simulink model "WindTurbine_FireProtection_System"  (R2024b)
settings: Solver=ode4  StartTime=0.0  StopTime=60  FixedStep=0.1  RelTol=1e-3
libraries: simulink x3
settings Model: Creator=LENOVO  LastModifiedBy=LENOVO

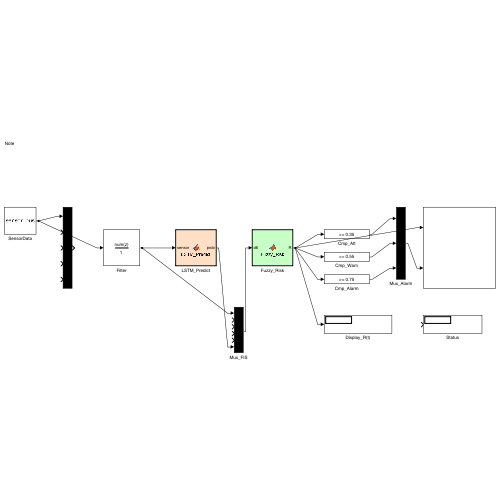
[thumbnail: Simulink's stored preview of the top-level diagram]
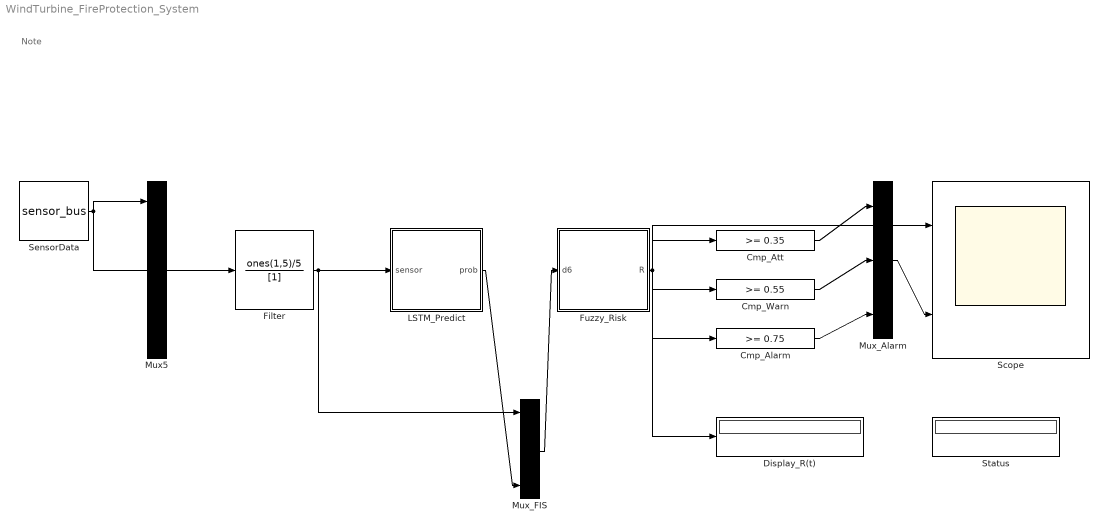
== system WindTurbine_FireProtection_System ==
  note: Note
  Cmp_Alarm : simulink/Logic and Bit Operations/Compare To Constant  relop=>=  const=0.75  OutDataTypeStr=boolean
  Cmp_Att : simulink/Logic and Bit Operations/Compare To Constant  relop=>=  const=0.35  OutDataTypeStr=boolean
  Cmp_Warn : simulink/Logic and Bit Operations/Compare To Constant  relop=>=  const=0.55  OutDataTypeStr=boolean
  Display_R(t) : Display
  Filter : DiscreteFilter  Numerator=ones(1,5)/5  Denominator=[1]  SampleTime=0.1
  Fuzzy_Risk : MATLAB Function  TreatAsAtomicUnit=on
  LSTM_Predict : MATLAB Function  TreatAsAtomicUnit=on
  Mux5 : Mux  Inputs=5
  Mux_Alarm : Mux  Inputs=3
  Mux_FIS : Mux  Inputs=6
  Scope : Scope  NumInputPorts=2
  SensorData : FromWorkspace  VariableName=sensor_bus
  Status : Display
  wires:
  SensorData/1 -> Mux5/1, Filter/1
  Filter/1 -> LSTM_Predict/1(sensor), Mux_FIS/1
  LSTM_Predict/1(prob) -> Mux_FIS/6
  Mux_FIS/1 -> Fuzzy_Risk/1(d6)
  Fuzzy_Risk/1(R) -> Cmp_Att/1, Cmp_Warn/1, Cmp_Alarm/1, Display_R(t)/1, Scope/1
  Cmp_Att/1 -> Mux_Alarm/1
  Cmp_Warn/1 -> Mux_Alarm/2
  Cmp_Alarm/1 -> Mux_Alarm/3
  Mux_Alarm/1 -> Scope/2

== matlab function WindTurbine_FireProtection_System/LSTM_Predict ==
  data: sensor input; prob output
function prob = LSTM_Predict(sensor)
persistent buf
if isempty(buf), buf = zeros(5,60); end
buf(:,1:59) = buf(:,2:60);
buf(:,60) = sensor(:);
prob = min(mean(buf(:,end-9:end),'all')*1.2, 0.95);
end

== matlab function WindTurbine_FireProtection_System/Fuzzy_Risk ==
  data: d6 input; R output
function R = Fuzzy_Risk(d6)
persistent fis
if isempty(fis)
    try; fis = readfis('WindTurbineFireRisk.fis'); catch; fis=[]; end
end
if ~isempty(fis)
    R = evalfis(fis, d6(:)');
else
    w = [0.18,0.16,0.16,0.12,0.08,0.30];
    R = sum(w .* d6(:)');
end
R = min(max(R,0),1);
end
